simulink model "prob_2"  (R2020b)
settings: Solver=VariableStepAuto  StartTime=0.0  StopTime=100  RelTol=1e-3
values from neighbouring files (symbols this model uses):
  b = 50    [prob_2matfile.m]
  k1 = 50    [prob_2matfile.m]
  k2 = 2000    [prob_2matfile.m]
  m1 = 100    [prob_2matfile.m]
  m2 = 5    [prob_2matfile.m]
settings Model: Creator=Akshay A H  LastModifiedBy=Akshay A H

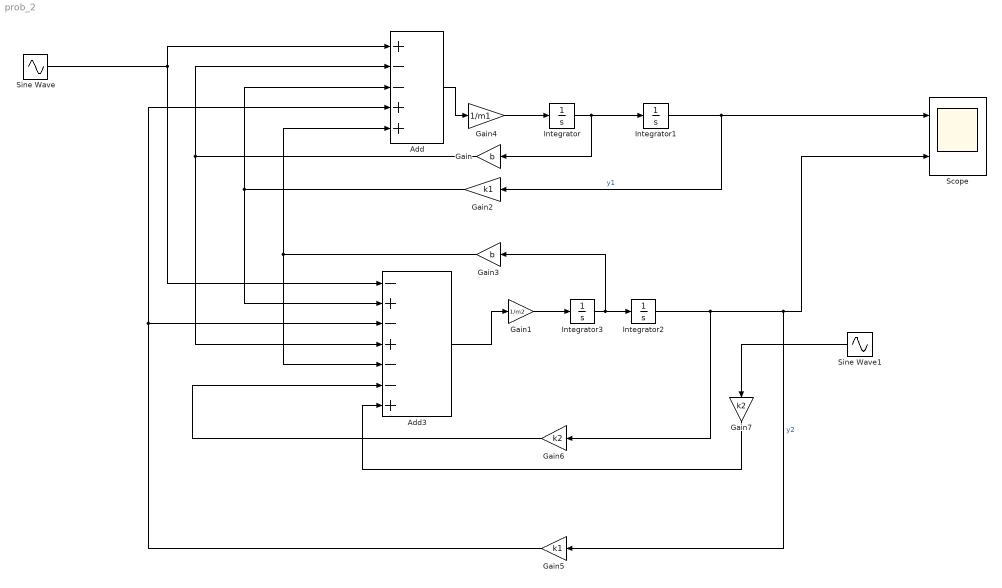
== system prob_2 ==
  Add : Sum  Inputs=+--++
  Add3 : Sum  Inputs=-+-+--+
  Gain : Gain  Gain=b
  Gain1 : Gain  Gain=1/m2
  Gain2 : Gain  Gain=k1
  Gain3 : Gain  Gain=b
  Gain4 : Gain  Gain=1/m1
  Gain5 : Gain  Gain=k1
  Gain6 : Gain  Gain=k2
  Gain7 : Gain  Gain=k2
  Integrator{,1..3} (4 alike) : Integrator
  Scope : Scope  NumInputPorts=2
  Sine Wave : Sin  Amplitude=2  Frequency=10  SampleTime=0
  Sine Wave1 : Sin  Amplitude=2  Frequency=10  SampleTime=0
  wires:
  Sine Wave1/1 -> Gain7/1
  Add3/1 -> Gain1/1
  Integrator2/1 -> Gain6/1, Scope/2, Gain5/1  "y2"
  Integrator3/1 -> Gain3/1, Integrator2/1
  Gain2/1 -> Add3/2, Add/3
  Gain4/1 -> Integrator/1
  Sine Wave/1 -> Add/1, Add3/1
  Gain/1 -> Add3/4, Add/2
  Add/1 -> Gain4/1
  Gain5/1 -> Add/4, Add3/3
  Gain3/1 -> Add3/5, Add/5
  Gain1/1 -> Integrator3/1
  Integrator/1 -> Gain/1, Integrator1/1
  Integrator1/1 -> Gain2/1, Scope/1  "y1"
  Gain6/1 -> Add3/6
  Gain7/1 -> Add3/7
